simulink model "pid_10"  (R2022a)
settings: Solver=FixedStepAuto  StartTime=0.0  StopTime=12.0  FixedStep=0.1  RelTol=1e-3  EnableMultiTasking=on
libraries: mbedblockslib x27, simulink x3, hdlsllib x2, slctrlblks x1, slpidlib x1
(part 2 of 2)

== stateflow chart pid_10/PID Tuning (ERROR)/Motor Ctrl/Motor_Ctrl ==
  state SHUTDOWN % Blower Off
    state Stop_1 % I2C to Anal.
      entry: mtr = 0;
      exit:
    state Stop_2 % Motor Brake
      entry:
      mtr_brk = 0; % Enable
      exit:
    state Stop_3 % Motor Disable
      entry:
      mtr_dis = 0; % Disable
      exit:
    state Stop_4 % Main Power
      entry:
      mtr_pwr = 0; % OFF
      exit:
    (default) -> Stop_1 % I2C to Anal.
    Stop_1 % I2C to Anal. -> Stop_2 % Motor Brake : after(1,sec)
    Stop_2 % Motor Brake -> Stop_3 % Motor Disable : after(500,msec)
    Stop_3 % Motor Disable -> Stop_4 % Main Power : after(1,sec)
  state STARTUP % Blower Start
    state Start_1 % Main Power
      entry:
      mtr_pwr = 0; % ON
      mtr_brk = 0; % Enabled
      mtr_dis = 0; % Disabled
      exit:
    (default) -> STARTUP.Start_1 % Main Power
  state Start_Mtr % Blower On
    state Start_1 % Main Power
      entry:
      mtr_pwr = 1; % ON
      exit:
    state Start_2 % Motor Brake
      entry:
      mtr_brk = 1; % Disable
      mtr_dis = 1; % Enabled
      exit:
    (default) -> Start_Mtr.Start_1 % Main Power
    Start_Mtr.Start_1 % Main Power -> Start_2 % Motor Brake : after(1,sec)
  state Run_Mtr % Continuous
    entry: mtr =1; % I2C output
    exit:
    note: Continuously Run the
        | Motor until Stop bit set
  note: Stop Motor after 3min
  note: Wait for Start
  note: POWER PIN:
      | Disable = <0.8V or Gnd
      | Enable = >30V or Not wired
  note: BRAKE PIN:
      | Enabled = <0.8V or Gnd
      | Deactivated = >2.4V or Not wired
  note: DISABLE PIN:
      | Disable = <0.8V or Gnd
      | Enable = >2.4V or Not wired
  note: 1. Power - On
      | 2. Brake - Off
      | 3. Disable - Off
      | 4. Voltage Output
  (default) -> STARTUP % Blower Start
  Run_Mtr % Continuous -> SHUTDOWN % Blower Off : after(5,sec)
  STARTUP % Blower Start -> (junction 53) : after(100,msec)
  (junction 53) -> Start_Mtr % Blower On [order 1] : [power == 1]
  (junction 53) -> STARTUP % Blower Start [order 2] : [power == 0]
  Start_Mtr % Blower On -> Run_Mtr % Continuous : after(2,sec)
  data: mtr output; mtr_brk output; mtr_pwr output; power input; mtr_dis output

== matlab function pid_10/Sensor & Motor/Motor Ctrl/Subsystem/MATLAB Function ==
  data: pwr input; mtr_ctrl output; user input; mtr_pwr output; mtr_brk output; press input; mtr_dis output
function [mtr_ctrl, mtr_pwr, mtr_brk, mtr_dis] = fcn(pwr, user, press)

if pwr >= 1
    mtr_pwr = 1;
    % delay()
    mtr_brk = 1;
    mtr_dis = 1;
else
    mtr_pwr = 0;
    % delay()
    mtr_brk = 0;
    mtr_dis = 0;
end

while user >= press
    speed += 1;         % needs initial value?
    mtr_ctrl = speed;   % update speed control I2C
end

== matlab function pid_10/Sensor & Motor/Motor Ctrl/Subsystem/MATLAB Function1 ==
  data: pwr input; mtr_pwr output; mtr_brk output; mtr_dis output
function [mtr_pwr, mtr_brk, mtr_dis] = fcn(pwr)

delay = 100;

% Enable all Motor Pins
if pwr >= 1
    mtr_pwr = 1;
    % delay()
    mtr_brk = 1;
    mtr_dis = 1;
% Disable all Motor Pins
else
    mtr_dis = 0;
    mtr_brk = 0;
    pause(delay);
    mtr_pwr = 0;
end

== matlab function pid_10/PID Tuning (ERROR)/Motor Ctrl/Subsystem/MATLAB Function1 ==
  data: pwr input; mtr_pwr output; mtr_brk output; mtr_dis output
function [mtr_pwr, mtr_brk, mtr_dis] = fcn(pwr)

delay = 100;

% Enable all Motor Pins
if pwr >= 1
    mtr_pwr = 1;
    % delay()
    mtr_brk = 1;
    mtr_dis = 1;
% Disable all Motor Pins
else
    mtr_dis = 0;
    mtr_brk = 0;
    pause(delay);
    mtr_pwr = 0;
end
